simulink model "max_pooling_int"  (R2024b)
settings: Solver=FixedStepDiscrete  StartTime=0.0  StopTime=10.0  RelTol=1e-3
InitFcn:
  | % Define a random matrix size between 3 and 10
  | n =6;
  | 
  | fprintf('Size of matrix A: n = %d\n', n);
libraries: simulink x1
settings Model: DataTypeOverride=Off  Creator=valen  LastModifiedBy=valen
settings SolverCC: AlgebraicLoopSolver=TrustRegion
settings DataIOCC: LimitDataPoints=on  SaveOutput=off  SaveTime=off
settings OptimizationCC: BlockReduction=off  ConditionallyExecuteInputs=off  DefaultParameterBehavior=Inlined  LifeSpan=inf
settings DebuggingCC: AlgebraicLoopMsg=error  SingleTaskRateTransMsg=error  UnconnectedInputMsg=warning  UnconnectedOutputMsg=warning  UnconnectedLineMsg=warning  AllowSymbolicDim=off  StrictBusMsg=ErrorOnBusTreatedAsVector  SFUnexpectedBacktrackingDiag=warning  SFNoUnconditionalDefaultTransitionDiag=warning  SFExecutionAtInitializationDiag=none  ArithmeticOperatorsInVariantConditions=warning
settings HardwareCC: ProdBitPerPointer=32  ProdBitPerSizeT=32  ProdBitPerPtrDiffT=32  ProdLargestAtomicFloat=None  ProdIntDivRoundTo=Undefined  ProdEndianess=Unspecified  ProdWordSize=32  ProdHWDeviceType=ASIC/FPGA->ASIC/FPGA  ProdEqTarget=off
settings ModelReferenceCC: EnableRefExpFcnMdlSchedulingChecks=on
settings SFSimCC: SimUseLocalCustomCode=off  CustomCodeUndefinedFunction=UseInterfaceOnly
settings RTWCC: RTWUseLocalCustomCode=off  GPUComputeCapability=3.5
settings CodeAppCC: StateflowObjectComments=on
settings GRTTargetCC: TargetLangStandard=C89/C90 (ANSI)
settings ConfigComp: CovScope=ReferencedModels  CovMetricSettings=dw  CovSaveCumulativeToWorkspaceVar=on  CovSaveSingleToWorkspaceVar=on  CovExternalEMLEnable=off  CovSFcnEnable=off

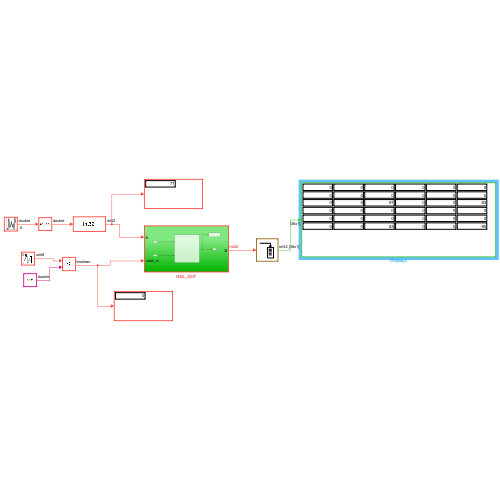
[thumbnail: Simulink's stored preview of the top-level diagram]
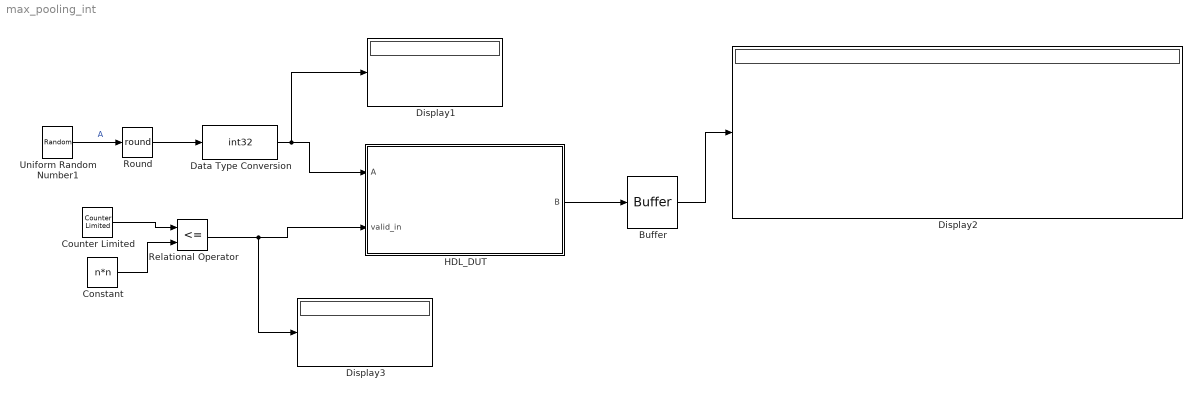
== system max_pooling_int ==
  Buffer : Buffer  N=n*n  OutputFrames=off
  Constant : Constant  Value=n*n
  Counter Limited : simulink/Sources/Counter Limited  uplimit=n*(n+1)  tsamp=-1
  Data Type Conversion : DataTypeConversion  OutDataTypeStr=int32  SaturateOnIntegerOverflow=off  RndMeth=Floor
  Display1 : Display
  Display2 : Display
  Display3 : Display
  HDL_DUT : Subsystem
  Relational Operator : RelationalOperator  Operator=<=  OutDataTypeStr=boolean  RndMeth=Simplest  InputSameDT=off
  Round : Rounding  Operator=round
  Uniform Random Number1 : UniformRandomNumber  Minimum=0  Maximum=100  Seed=n  SampleTime=10/(n*n+1)
  wires:
  HDL_DUT/1(B) -> Buffer/1
  Constant/1 -> Relational Operator/2
  Uniform Random Number1/1 -> Round/1  "A"
  Counter Limited/1 -> Relational Operator/1
  Data Type Conversion/1 -> Display1/1, HDL_DUT/1(A)
  Relational Operator/1 -> Display3/1, HDL_DUT/2(valid_in)
  Buffer/1 -> Display2/1
  Round/1 -> Data Type Conversion/1

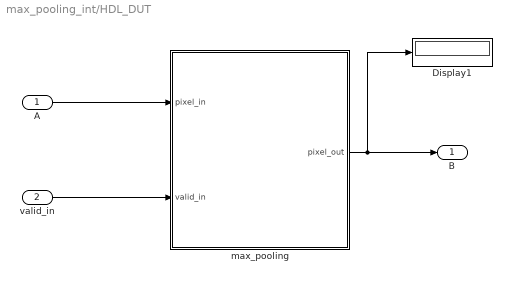
== system max_pooling_int/HDL_DUT ==
  A : Inport
  valid_in : Inport  Port=2
  Display1 : Display
  max_pooling : MATLAB Function  TreatAsAtomicUnit=on
  B : Outport  VectorParamsAs1DForOutWhenUnconnected=off
  wires:
  A/1 -> max_pooling/1(pixel_in)
  valid_in/1 -> max_pooling/2(valid_in)
  max_pooling/1(pixel_out) -> B/1, Display1/1

== matlab function max_pooling_int/HDL_DUT/max_pooling ==
  data: pixel_in input; pixel_out output; valid_in input
function pixel_out  = hardware_max_pooling(pixel_in, valid_in)
 % Configuration
 SIZE = 6; % Largeur de l'image (10x10 = 100 pixels au total)
 STRIDE = 3; % Fenêtre 2x2, Stride 2

 % Nombre de blocs de pooling à stocker horizontalement
 NUM_BLOCKS_X = SIZE / STRIDE;
 
 % Le line_buffer stocke le maximum temporaire de chaque colonne (taille 10)
 persistent line_buffer count;
 if isempty(count)
    line_buffer    = zeros(1, NUM_BLOCKS_X, 'int32');
    count          = int32(0);
 end
 
 % Signaux de sortie par défaut
 pixel_out = int32(0);
 
 if valid_in
    % 1. Détermination des coordonnées spatiales (0 à SIZE-1)
    curr_y = floor(single(count) / SIZE);
    curr_x = mod(single(count), SIZE);
 
    % Convertir l'index X pour MATLAB (1 à SIZE)
    idx_x = int32(floor(curr_x / STRIDE)) + 1;
 
    max_bloc_2d = max(line_buffer(idx_x), pixel_in);
 
    % On met à jour la RAM avec le nouveau max pour cette colonne
    line_buffer(idx_x) = max_bloc_2d;
 
     % 4. Transmission à la sortie et réinitialisation (Fin du Stride)
     % On est sur la dernière ligne du bloc ET la dernière colonne du bloc ?
    if mod(curr_y, STRIDE) == (STRIDE - 1) && mod(curr_x, STRIDE) == (STRIDE - 1)
 	        pixel_out = line_buffer(idx_x) ;
	        line_buffer(idx_x) = int32(0);
    end
              
    % Incrémentation du compteur global
    if count == int32(SIZE * SIZE - 1)
        count = int32(0);
    else
        count = count + 1;
    end
 end
end
